simulink model "acquire_data"  (R2021a)
settings: Solver=VariableStepAuto  StartTime=0.0  StopTime=1000.0  RelTol=1e-3
libraries: instrumentseriallib x2, mspfiltlib x1, sharedtransform x1
settings Model: SimulationMode=accelerator  Creator=maxab  LastModifiedBy=maxab

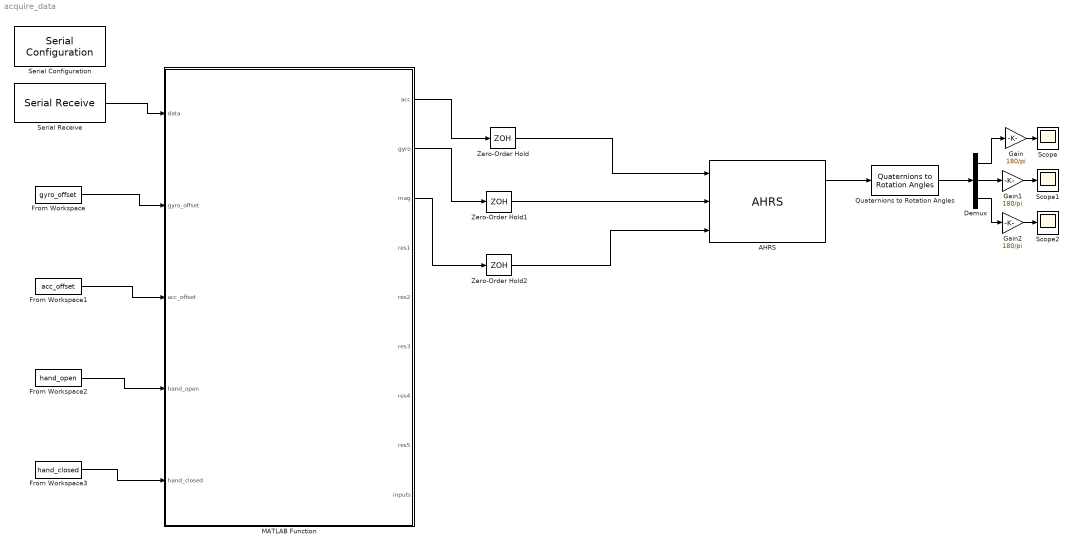
== system acquire_data ==
  AHRS : mspfiltlib/AHRS  DispRefFrame=NED  DecimationFactor=1  InitialProcessNoise=ahrsfilter.defaultProcessNoise  OrientationFormat=quaternion  SimulateUsing=Code generation  AccelerometerNoise=0.0001924722  GyroscopeNoise=9.1385e-5  MagnetometerNoise=0.1  GyroscopeDriftNoise=3.0462e-13  LinearAccelerationNoise=0.0096236100000000012  MagneticDisturbanceNoise=0.5  LinearAccelerationDecayFactor=0.5  MagneticDisturbanceDecayFactor=0.5  ExpectedMagneticFieldStrength=80
      settings: SourceProductBaseCode=TF,NV
  Demux : Demux  Outputs=3
  From Workspace : FromWorkspace  VariableName=gyro_offset
  From Workspace1 : FromWorkspace  VariableName=acc_offset
  From Workspace2 : FromWorkspace  VariableName=hand_open
  From Workspace3 : FromWorkspace  VariableName=hand_closed
  Gain : Gain  Gain=180/pi
  Gain1 : Gain  Gain=180/pi
  Gain2 : Gain  Gain=180/pi
  MATLAB Function : MATLAB Function  TreatAsAtomicUnit=on
  Quaternions to Rotation Angles : sharedtransform/Quaternions to Rotation Angles  rotationOrder=ZYX  aMode=aMode
      settings: SourceProductBaseCode=AE,PW,DR,MT,UV,VE
  Scope : Scope
  Scope1 : Scope
  Scope2 : Scope
  Serial Configuration : instrumentseriallib/Serial Configuration  Priority=-200000  Port=COM7  ComPort=COM7  BaudRate=38400  DataBits=8  Parity=none  StopBits=1  ByteOrder=little-endian  FlowControl=none  Timeout=10  SimulateUsing=Interpreted execution  BlockInModel=on
  Serial Receive : instrumentseriallib/Serial Receive  Priority=1  Port=COM7  ComPort=COM7  DataType=int16  SaveDataType=uint8  ToggleHeader=on  Header=[0xCA 0xFE]  ToggleTerminator=off  Terminator=<none>  CustomTerminator=[]  ToggleDataSize=on  DataSize=[13]  EnableBlockingMode=on  ActionDataUnavailable=Output last received value  ActionWhenDataUnavailable=Output last received value  CustomValue=0  SampleTime=0.05  SimulateUsing=Interpreted execution  BlockInModel=on
  Zero-Order Hold : ZeroOrderHold  SampleTime=0.05
  Zero-Order Hold1 : ZeroOrderHold  SampleTime=0.05
  Zero-Order Hold2 : ZeroOrderHold  SampleTime=0.05
  wires:
  Serial Receive/1 -> MATLAB Function/1(data)
  From Workspace/1 -> MATLAB Function/2(gyro_offset)
  From Workspace1/1 -> MATLAB Function/3(acc_offset)
  From Workspace2/1 -> MATLAB Function/4(hand_open)
  From Workspace3/1 -> MATLAB Function/5(hand_closed)
  Quaternions to Rotation Angles/1 -> Demux/1
  Demux/1 -> Gain/1
  Demux/2 -> Gain1/1
  MATLAB Function/1(acc) -> Zero-Order Hold/1
  MATLAB Function/2(gyro) -> Zero-Order Hold1/1
  MATLAB Function/3(mag) -> Zero-Order Hold2/1
  Demux/3 -> Gain2/1
  Gain/1 -> Scope/1
  Gain1/1 -> Scope1/1
  Gain2/1 -> Scope2/1
  Zero-Order Hold/1 -> AHRS/1
  Zero-Order Hold1/1 -> AHRS/2
  Zero-Order Hold2/1 -> AHRS/3
  AHRS/1 -> Quaternions to Rotation Angles/1

== matlab function acquire_data/MATLAB Function ==
  data: acc output; gyro output; mag output; data input; gyro_offset input; acc_offset input; hand_open input; hand_closed input; res1 output; res2 output; res3 output; res4 output; res5 output; inputs output
function [acc, gyro, mag, res1, res2, res3, res4, res5, inputs] = fcn(data, gyro_offset, acc_offset, hand_open, hand_closed)
    usb_data = data';
    
    gyro_offset = double(gyro_offset');
    acc_offset = double(acc_offset');
    hand_open = double(hand_open');
    hand_closed = double(hand_closed');
        
    gyro = double(usb_data(4:6)) * (2000 * pi / (180 * 2^15)) - gyro_offset; % rad/s
    acc = double(usb_data(1:3)) * 2 * 9.81 / (2^15) - acc_offset; % g-forces
    acc(3) = acc(3) * -1;
    mag = double(usb_data(10:12)) * 4 * 100 / (2^15); % microT
    
    res = [0 0 0 0 0];
    res(1) = bitand(uint16(usb_data(8)), uint16(hex2dec('00FF')), 'uint16');
    res(2) = bitand(typecast(uint16(usb_data(8)), 'uint16'), uint16(hex2dec('FF00')), 'uint16');
    res(2) = bitshift(uint16(usb_data(8)), -8, 'uint16'); % shift upper bits to lower place
    res(3) = bitand(uint16(usb_data(9)), uint16(hex2dec('00FF')), 'uint16');
    res(4) = bitand(typecast(uint16(usb_data(9)), 'uint16'), uint16(hex2dec('FF00')), 'uint16');
    res(4) = bitshift(uint16(usb_data(9)), -8, 'uint16'); % shift upper bits to lower place
    res(5) = bitand(uint16(usb_data(10)), uint16(hex2dec('00FF')), 'uint16');
    
    norm_res = [0 0 0 0 0];
    for res_index=1:5
        norm_res(res_index) = (res(res_index) - hand_open(res_index)) * 200 / (hand_closed(res_index) - hand_open(res_index));
    end
    
    res1 = norm_res(1);
    res2 = norm_res(2);
    res3 = norm_res(3);
    res4 = norm_res(4);
    res5 = norm_res(5);
    
    inputs = bitand(int16(usb_data(10)), int16(hex2dec('FF00')), 'int16');
    inputs = bitshift(int16(inputs), -8, 'int16'); % shift upper bits to lower place

end
